simulink model "harmonic_generating_load_Simulink"  (R2020b)
settings: Solver=ode23tb  StartTime=0.0  StopTime=0.1  MaxStep=5e-5  RelTol=1e-3
PreLoadFcn:
  | a=0
libraries: powerlib x11, powerlib_meascontrol x7, simulink x2
settings Model: Creator=acer  LastModifiedBy=Pchan
settings DataIOCC: ReturnWorkspaceOutputs=off
settings DebuggingCC: ArithmeticOperatorsInVariantConditions=warning
settings SFSimCC: SimUseLocalCustomCode=off  CustomCodeUndefinedFunction=UseInterfaceOnly
settings RTWCC: RTWUseLocalCustomCode=off
settings CodeAppCC: StateflowObjectComments=on
settings SimscapeCC: SimscapeNormalizeSystem=off

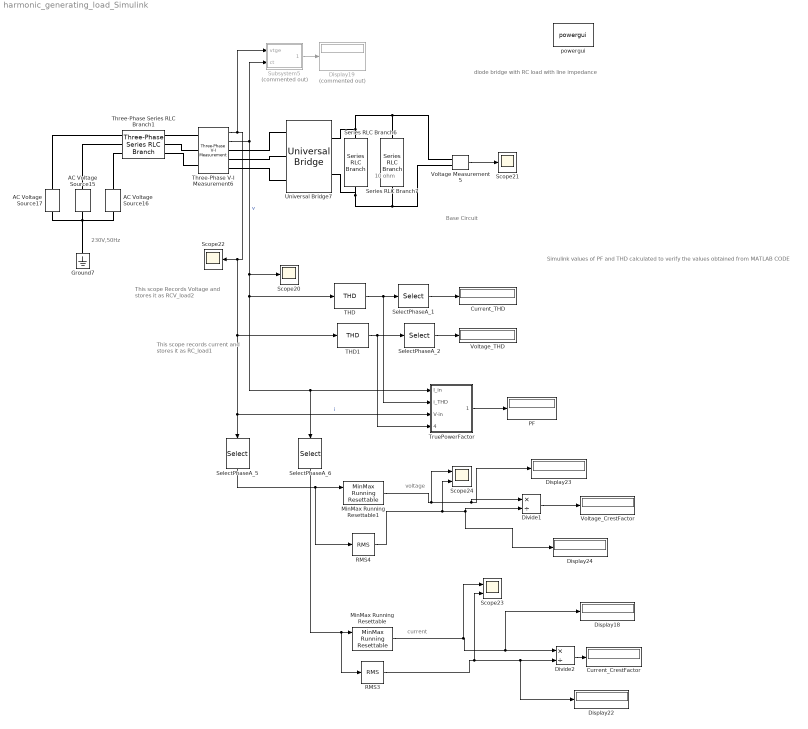
== system harmonic_generating_load_Simulink ==
  note: Base Circuit
  note: Simulink values of PF and THD calculated to verify the values obtained from MATLAB CODE
  note: This scope records current
      | and stores it as
      | RC_load1
  note: This scope Records Voltage and stores it as
      | RCV_load2
  note: voltage
  note: current
  note: 230V,50Hz
  note: 10 ohm
  note: diode bridge with RC load with line impedance
  AC Voltage Source15 : powerlib/Electrical Sources/AC Voltage Source  Amplitude=230*sqrt(2)  Phase=-120  Frequency=50  SampleTime=0  Measurements=None  BusType=swing  Pref=10e3  Qref=0  Qmin=-inf  Qmax=+inf
  AC Voltage Source16 : powerlib/Electrical Sources/AC Voltage Source  Amplitude=230*sqrt(2)  Phase=-240  Frequency=50  SampleTime=0  Measurements=None  BusType=swing  Pref=10e3  Qref=0  Qmin=-inf  Qmax=+inf
  AC Voltage Source17 : powerlib/Electrical Sources/AC Voltage Source  Amplitude=230*sqrt(2)  Phase=0  Frequency=50  SampleTime=0  Measurements=None  BusType=swing  Pref=10e3  Qref=0  Qmin=-inf  Qmax=+inf
  Current_CrestFactor : Display
  Current_THD : Display
  Display{18,22..24} (4 alike) : Display
  Display19 : Display  Commented=on
  Divide1 : Product  Inputs=*/
  Divide2 : Product  Inputs=*/
  Ground7 : powerlib/Elements/Ground  LConnTagsString=a
  MinMax Running Resettable : simulink/Math Operations/MinMax Running Resettable  Function=max  vinit=0.0
  MinMax Running Resettable1 : simulink/Math Operations/MinMax Running Resettable  Function=max  vinit=0.0
  PF : Display
  RMS3 : powerlib_meascontrol/Measurements/RMS  TrueRMS=off  Freq=50  RMSInit=0  Ts=0
  RMS4 : powerlib_meascontrol/Measurements/RMS  TrueRMS=on  Freq=50  RMSInit=0  Ts=0
  Scope20 : Scope
  Scope21 : Scope
  Scope22 : Scope
  Scope23 : Scope  NumInputPorts=2
  Scope24 : Scope  NumInputPorts=2
  SelectPhaseA_{1..2,5..6} (4 alike) : Selector  InputPortWidth=3  IndexOptions=Index vector (dialog)  Indices=1  OutputSizes=1
  Series RLC Branch6 : powerlib/Elements/Series RLC Branch  LConnTagsString=__new0  RConnTagsString=__new0  BranchType=R  Resistance=1  Inductance=1e-3  SetiL0=off  InitialCurrent=0  Capacitance=1e-6  Setx0=off  InitialVoltage=0  Measurements=None
  Series RLC Branch7 : powerlib/Elements/Series RLC Branch  LConnTagsString=__new0  RConnTagsString=__new0  BranchType=C  Resistance=5  Inductance=1e-3  SetiL0=off  InitialCurrent=0  Capacitance=5e-3  Setx0=off  InitialVoltage=0  Measurements=None
  Subsystem5 : Subsystem  Commented=on
  THD : powerlib_meascontrol/Measurements/THD  Freq=50  Ts=0
  THD1 : powerlib_meascontrol/Measurements/THD  Freq=50  Ts=0
  Three-Phase Series RLC Branch1 : powerlib/Elements/Three-Phase Series RLC Branch  LConnTagsString=A|B|C  RConnTagsString=A|B|C  BranchType=RL  Resistance=0.86  Inductance=0.01e-6  Capacitance=1e-6  Measurements=None
  Three-Phase V-I Measurement6 : powerlib/Measurements/Three-Phase V-I Measurement  VoltageMeasurement=phase-to-ground  SetLabelV=off  LabelV=Vabc  Vpu=off  VpuLL=off  CurrentMeasurement=yes  SetLabelI=off  LabelI=Iabc  Ipu=off  Pbase=100e6  Vbase=500e3  OutputType=Complex  PhasorSimulation=off  PSBequivalent=0
  TruePowerFactor : Subsystem
  Universal Bridge7 : powerlib/Power Electronics/Universal Bridge  Arms=3  SnubberResistance=1e5  SnubberCapacitance=inf  Device=Diodes  Ron=1e-3  Lon=0  ForwardVoltages="[  0  0  ]"  ForwardVoltage=0  GTOparameters=[ 10e-6 , 20e-6 ]  IGBTparameters=[ 1e-6 , 2e-6 ]  Measurements=None  Measurements_2=None  converterType=Rectifier
  Voltage Measurement5 : powerlib/Measurements/Voltage Measurement  PhasorSimulation=off  OutputType=Complex  PSBequivalent=0
  Voltage_CrestFactor : Display
  Voltage_THD : Display
  powergui : powerlib/powergui  Priority=1  SimulationMode=Discrete  SampleTime=5e-7  frequency=60  Iterations=50  frequencyindice=0  Pbase=100e6  ErrMax=1e-4  UnitsV=kV  UnitsW=MW  buscounter=0  FunctionMessages=off  echomessages=off  EnableUseOfTLC=off  CurrentSourceSwitches=off  DisableSnubberDevices=off  DisableRonSwitches=off  DisableVfSwitches=off  DisplayEquations=off  AutomaticDiscreteSolvers=off  SolverType=Backward Euler  Interpol=off  ExternalGateDelay=off  methode=off  Ts=10  x0status=blocks  SPID=off  SwTol=0  HookPort=off  NonlinearTolerance=1e-4  nMaxIteration=100  ContinueOnMaxIteration=off  RestoreLinks=warning  ResistiveCurrentMeasurement=off  Frange=[0:2:500]  Ylog=off  Xlog=on  ShowGrid=off  save=off  variable=ZData  structure=Invload4  ZoomFFT=off  StartTime=0  cycles=5  DisplayStyle=4  fundamental=50  FreqAxis=off  MaxFrequency=5000  frequencyindicesteady=1  RmsSteady=1  display=off
  wires:
  Voltage Measurement5/1 -> Scope21/1
  Subsystem5/1(power) -> Display19/1
  THD/1 -> TruePowerFactor/2(i_THD), SelectPhaseA_1/1
  THD1/1 -> TruePowerFactor/4(v_THD), SelectPhaseA_2/1
  SelectPhaseA_1/1 -> Current_THD/1
  SelectPhaseA_2/1 -> Voltage_THD/1
  TruePowerFactor/1(TruePF) -> PF/1
  Three-Phase V-I Measurement6/1 -> Subsystem5/1(vtge), TruePowerFactor/3(V-in), SelectPhaseA_5/1, THD1/1, Scope22/1  "i"
  RMS4/1 -> Display24/1, Divide1/2, Scope24/2
  Divide2/1 -> Current_CrestFactor/1
  MinMax Running Resettable1/1 -> Scope24/1, Display23/1, Divide1/1
  MinMax Running Resettable/1 -> Scope23/1, Display18/1, Divide2/1
  RMS3/1 -> Display22/1, Divide2/2, Scope23/2
  Divide1/1 -> Voltage_CrestFactor/1
  Three-Phase V-I Measurement6/2 -> TruePowerFactor/1(I_in), SelectPhaseA_6/1, THD/1, Scope20/1, Subsystem5/2(ct)  "v"
  SelectPhaseA_6/1 -> MinMax Running Resettable/1, RMS3/1
  SelectPhaseA_5/1 -> MinMax Running Resettable1/1, RMS4/1
  connections:
  Ground7/LConn1 -- AC Voltage Source15/LConn1 -- AC Voltage Source16/LConn1 -- AC Voltage Source17/LConn1
  Universal Bridge7/RConn1 -- Voltage Measurement5/LConn1 -- Series RLC Branch7/LConn1 -- Series RLC Branch6/LConn1
  Series RLC Branch6/RConn1 -- Universal Bridge7/RConn2 -- Voltage Measurement5/LConn2 -- Series RLC Branch7/RConn1
  Three-Phase V-I Measurement6/RConn2 -- Universal Bridge7/LConn2
  Three-Phase V-I Measurement6/RConn3 -- Universal Bridge7/LConn3
  Universal Bridge7/LConn1 -- Three-Phase V-I Measurement6/RConn1
  Three-Phase Series RLC Branch1/RConn1 -- Three-Phase V-I Measurement6/LConn1
  Three-Phase Series RLC Branch1/RConn2 -- Three-Phase V-I Measurement6/LConn2
  Three-Phase Series RLC Branch1/RConn3 -- Three-Phase V-I Measurement6/LConn3
  Three-Phase Series RLC Branch1/LConn1 -- AC Voltage Source17/RConn1
  Three-Phase Series RLC Branch1/LConn2 -- AC Voltage Source15/RConn1
  Three-Phase Series RLC Branch1/LConn3 -- AC Voltage Source16/RConn1

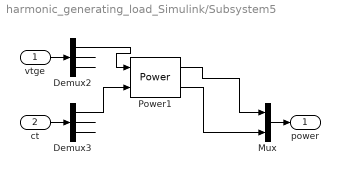
== system harmonic_generating_load_Simulink/Subsystem5 ==
  vtge : Inport
  ct : Inport  Port=2
  Demux2 : Demux  Outputs=3
  Demux3 : Demux  Outputs=3
  Mux : Mux  Inputs=2
  Power1 : powerlib_meascontrol/Measurements/Power  Freq=50  Vinit=[1, 0]  Iinit=[1, 0]  Ts=0
  power : Outport
  wires:
  Demux2/1 -> Power1/1
  Demux3/1 -> Power1/2
  Power1/2 -> Mux/2
  Power1/1 -> Mux/1
  Demux3/2 -> ?
  Demux3/3 -> ?
  vtge/1 -> Demux2/1
  Demux2/2 -> ?
  Demux2/3 -> ?
  ct/1 -> Demux3/1
  Mux/1 -> power/1

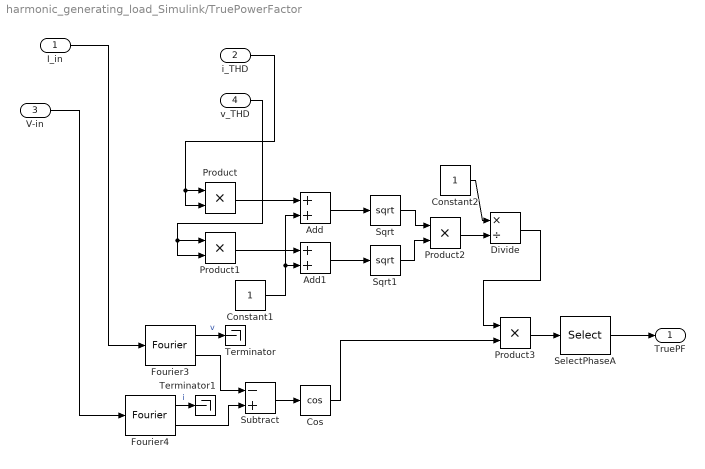
== system harmonic_generating_load_Simulink/TruePowerFactor ==
  I_in : Inport
  i_THD : Inport  Port=2
  V-in : Inport  Port=3
  v_THD : Inport  Port=4
  Add : Sum
  Add1 : Sum
  Constant1 : Constant
  Constant2 : Constant
  Cos : Trigonometry  Operator=cos
  Divide : Product  Inputs=*/
  Fourier3 : powerlib_meascontrol/Measurements/Fourier  Freq=50  n=1  InInit=[0, 0]  Ts=0
  Fourier4 : powerlib_meascontrol/Measurements/Fourier  Freq=50  n=1  InInit=[0, 0]  Ts=0
  Product{,1..3} (4 alike) : Product
  SelectPhaseA : Selector  InputPortWidth=3  IndexOptions=Index vector (dialog)  Indices=1  OutputSizes=1
  Sqrt : Sqrt  SaturateOnIntegerOverflow=on
  Sqrt1 : Sqrt  SaturateOnIntegerOverflow=on
  Subtract : Sum  Inputs=-+
  Terminator : Terminator
  Terminator1 : Terminator
  TruePF : Outport
  wires:
  Product1/1 -> Add1/1
  Divide/1 -> Product3/1
  i_THD/1 -> Product/2, Product/1
  Product3/1 -> SelectPhaseA/1
  SelectPhaseA/1 -> TruePF/1
  Add1/1 -> Sqrt1/1
  Product/1 -> Add/1
  v_THD/1 -> Product1/2, Product1/1
  Constant1/1 -> Add1/2, Add/2
  Sqrt1/1 -> Product2/2
  Product2/1 -> Divide/2
  Constant2/1 -> Divide/1
  Cos/1 -> Product3/2
  Fourier3/2 -> Subtract/1
  Subtract/1 -> Cos/1
  Sqrt/1 -> Product2/1
  Fourier4/2 -> Subtract/2
  Add/1 -> Sqrt/1
  I_in/1 -> Fourier3/1
  V-in/1 -> Fourier4/1
  Fourier3/1 -> Terminator/1  "v"
  Fourier4/1 -> Terminator1/1  "i"
